simulink model "CommandLimits"  (R2017b)
settings: configuration reference "Autosar_CodeGeneration" (kept outside this file)
settings Model: RequirementInfo={'linktype_rmi_url' 'http://md1hxhhc.ww004.siemens.net/polarion/' '@/project/ATRover/workitem?id=ATR-529' 'true' 'Polarion: ATR-529' '' ; 'linktype_rmi_url' 'http://md1hxhhc.ww004.siemens.net/polarion/' '@/project/ATRover/workitem?id=ATR-594' 'true' 'Polarion: ATR-594' '' } %GIDa_e2c0a0a6_deb1_4459_85d0_b00cc8d3b9da  DataDictionary=RoverDataDict.sldd  Creator=zwqe6u  LastModifiedBy=eh6qym
settings ConfigSetRef: DDName=RoverDataDict.sldd

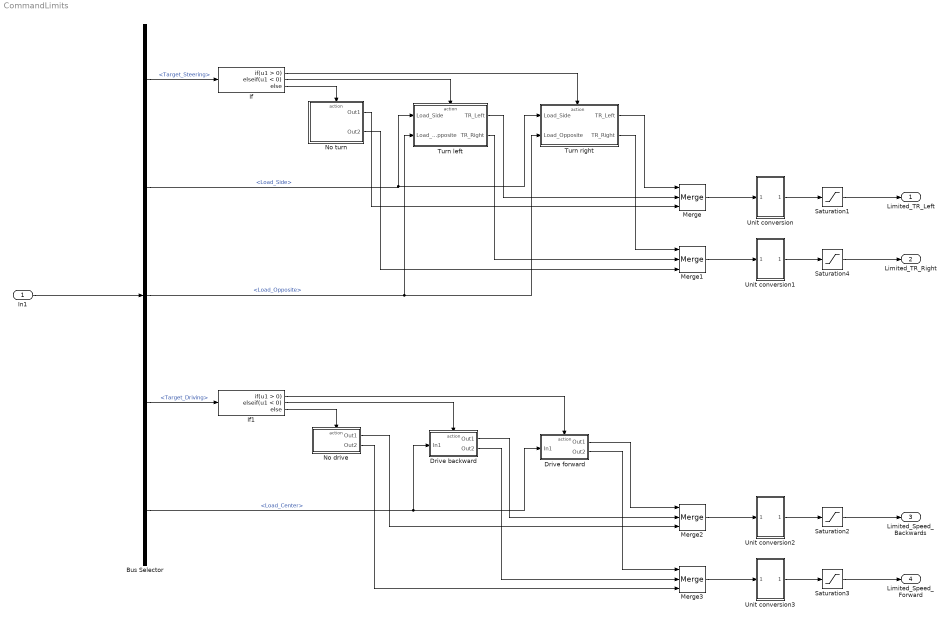
== system CommandLimits ==
  In1 : Inport  OutDataTypeStr=Bus: Obstacle_Detection_Out
  Bus Selector : BusSelector  OutputSignals=Target_Steering,Load_Side,Load_Opposite,Target_Driving,Load_Center
  Drive backward : Subsystem  TreatAsAtomicUnit=on
  Drive forward : Subsystem  TreatAsAtomicUnit=on
  If : If  ElseIfExpressions=u1 < 0
  If1 : If  ElseIfExpressions=u1 < 0
  Merge : Merge  Inputs=3  InitialOutput=[-1]
  Merge1 : Merge  Inputs=3  InitialOutput=[1]
  Merge2 : Merge  Inputs=3  InitialOutput=[-1]
  Merge3 : Merge  Inputs=3  InitialOutput=[1]
  No drive : Subsystem  TreatAsAtomicUnit=on
  No turn : Subsystem  TreatAsAtomicUnit=on
  Saturation1 : Saturate  UpperLimit=5  LowerLimit=0
  Saturation2 : Saturate  UpperLimit=2.5  LowerLimit=0
  Saturation3 : Saturate  UpperLimit=5  LowerLimit=2.5
  Saturation4 : Saturate  UpperLimit=5  LowerLimit=0
  Turn left : Subsystem  TreatAsAtomicUnit=on
  Turn right : Subsystem  TreatAsAtomicUnit=on
  Unit conversion : Subsystem
  Unit conversion1 : Subsystem
  Unit conversion2 : Subsystem
  Unit conversion3 : Subsystem
  Limited_TR_Left : Outport  OutDataTypeStr=double
  Limited_TR_Right : Outport  Port=2  OutDataTypeStr=double
  Limited_Speed_Backwards : Outport  Port=3  OutDataTypeStr=double
  Limited_Speed_Forward : Outport  Port=4  OutDataTypeStr=double
  wires:
  In1/1 -> Bus Selector/1
  Drive forward/1(Out1) -> Merge2/1
  Drive backward/1(Out1) -> Merge2/2
  Drive forward/2(Out2) -> Merge3/1
  Drive backward/2(Out2) -> Merge3/2
  Unit conversion2/1(Out1) -> Saturation2/1
  Unit conversion3/1(Out1) -> Saturation3/1
  Bus Selector/4 -> If1/1  "<Target_Driving>"
  If1/1 -> Drive forward/Action
  If1/2 -> Drive backward/Action
  Merge1/1 -> Unit conversion1/1(In1)
  Merge/1 -> Unit conversion/1(In1)
  Merge2/1 -> Unit conversion2/1(In1)
  Merge3/1 -> Unit conversion3/1(In1)
  Unit conversion/1(Out1) -> Saturation1/1
  Unit conversion1/1(Out1) -> Saturation4/1
  Saturation2/1 -> Limited_Speed_Backwards/1
  Saturation3/1 -> Limited_Speed_Forward/1
  Saturation1/1 -> Limited_TR_Left/1
  Saturation4/1 -> Limited_TR_Right/1
  If1/3 -> No drive/Action
  No drive/1(Out1) -> Merge2/3
  No drive/2(Out2) -> Merge3/3
  Bus Selector/5 -> Drive forward/1(In1), Drive backward/1(In1)  "<Load_Center>"
  Bus Selector/3 -> Turn right/2(Load_Opposite), Turn left/2(Load_Opposite)  "<Load_Opposite>"
  Bus Selector/2 -> Turn right/1(Load_Side), Turn left/1(Load_Side)  "<Load_Side>"
  Turn right/1(TR_Left) -> Merge/1
  Turn right/2(TR_Right) -> Merge1/1
  If/1 -> Turn right/Action
  If/2 -> Turn left/Action
  Turn left/1(TR_Left) -> Merge/2
  Turn left/2(TR_Right) -> Merge1/2
  If/3 -> No turn/Action
  No turn/1(Out1) -> Merge/3
  No turn/2(Out2) -> Merge1/3
  Bus Selector/1 -> If/1  "<Target_Steering>"

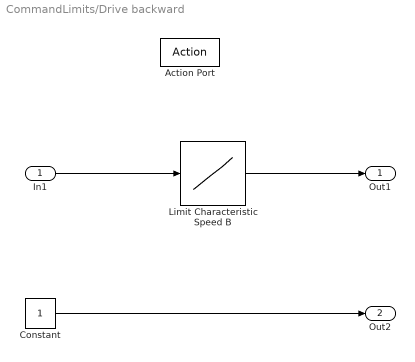
== system CommandLimits/Drive backward ==
  In1 : Inport
  Action Port : ActionPort  ActionType=elseif
  Constant : Constant
  Limit Characteristic Speed B : Lookup_n-D  NumberOfTableDimensions=1  BreakpointsForDimension1=[0.06 0.10 0.30 0.80]  Table=[0 0 -0.1 -1]  RemoveProtectionInput=on  InternalRulePriority=Speed  RndMeth=Simplest  InputSameDT=on
  Out1 : Outport  InitialOutput=[-1]
  Out2 : Outport  Port=2  InitialOutput=[1]
  wires:
  Limit Characteristic Speed B/1 -> Out1/1
  In1/1 -> Limit Characteristic Speed B/1
  Constant/1 -> Out2/1

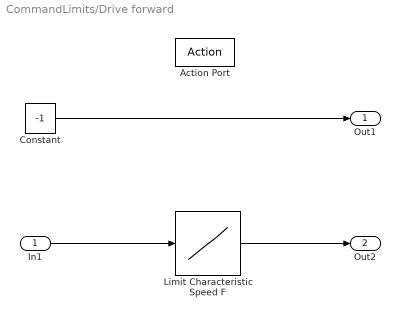
== system CommandLimits/Drive forward ==
  In1 : Inport
  Action Port : ActionPort  ActionType=then
  Constant : Constant  Value=-1
  Limit Characteristic Speed F : Lookup_n-D  NumberOfTableDimensions=1  BreakpointsForDimension1=[0.06 0.10 0.30 0.80]  Table=[0 0 0.1 1]  RemoveProtectionInput=on  InternalRulePriority=Speed  RndMeth=Simplest  InputSameDT=on
  Out1 : Outport  InitialOutput=[-1]
  Out2 : Outport  Port=2  InitialOutput=[1]
  wires:
  Limit Characteristic Speed F/1 -> Out2/1
  In1/1 -> Limit Characteristic Speed F/1
  Constant/1 -> Out1/1

== system CommandLimits/No drive ==
  Action Port : ActionPort  ActionType=else
  Constant : Constant  Value=-1
  Constant1 : Constant
  Out1 : Outport  InitialOutput=[0.8]
  Out2 : Outport  Port=2  InitialOutput=[0.8]
  wires:
  Constant/1 -> Out1/1
  Constant1/1 -> Out2/1

== system CommandLimits/No turn ==
  Action Port : ActionPort  ActionType=else
  Constant : Constant  Value=-1
  Constant1 : Constant
  Out1 : Outport  InitialOutput=[-1]
  Out2 : Outport  Port=2  InitialOutput=[1]
  wires:
  Constant/1 -> Out1/1
  Constant1/1 -> Out2/1

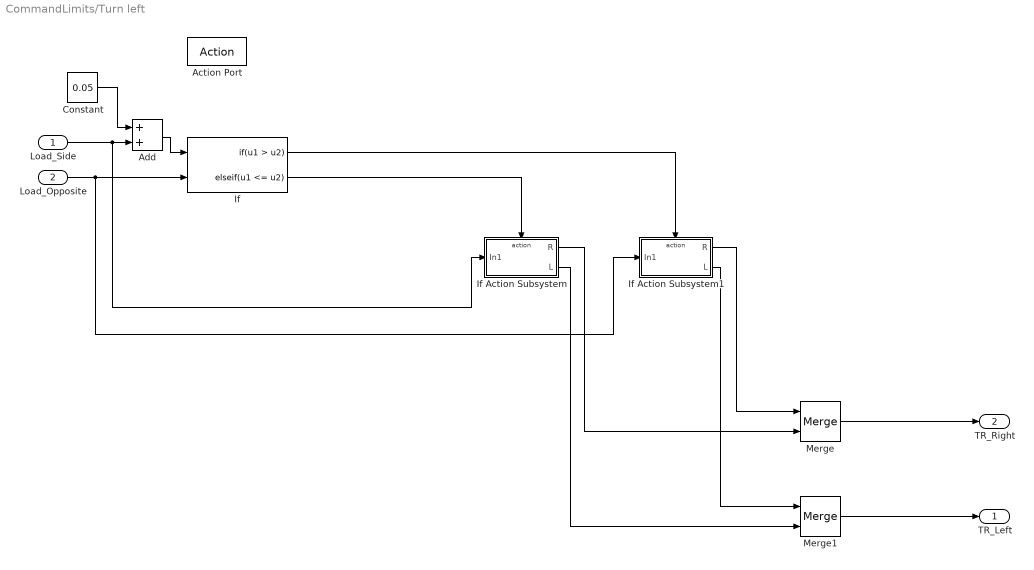
== system CommandLimits/Turn left ==
  Load_Side : Inport
  Load_Opposite : Inport  Port=2
  Action Port : ActionPort  ActionType=elseif
  Add : Sum
  Constant : Constant  Value=0.05
  If : If  NumInputs=2  IfExpression=u1 > u2  ElseIfExpressions=u1 <= u2  ShowElse=off
  If Action Subsystem : Subsystem  TreatAsAtomicUnit=on
  If Action Subsystem1 : Subsystem  TreatAsAtomicUnit=on
  Merge : Merge  InitialOutput=[1]
  Merge1 : Merge  InitialOutput=[-1]
  TR_Left : Outport  InitialOutput=[-1]
  TR_Right : Outport  Port=2  InitialOutput=[1]
  wires:
  Load_Opposite/1 -> If/2, If Action Subsystem1/1(In1)
  If Action Subsystem1/1(R) -> Merge/1
  If Action Subsystem/1(R) -> Merge/2
  If/1 -> If Action Subsystem1/Action
  If Action Subsystem/2(L) -> Merge1/2
  If Action Subsystem1/2(L) -> Merge1/1
  Load_Side/1 -> If Action Subsystem/1(In1), Add/2
  Merge1/1 -> TR_Left/1
  Merge/1 -> TR_Right/1
  If/2 -> If Action Subsystem/Action
  Constant/1 -> Add/1
  Add/1 -> If/1

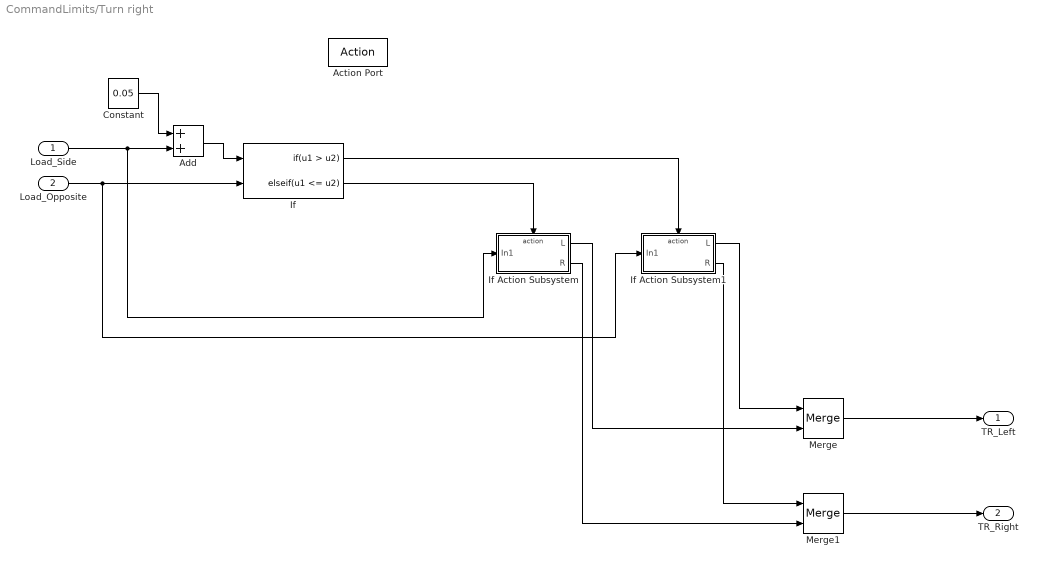
== system CommandLimits/Turn right ==
  Load_Side : Inport
  Load_Opposite : Inport  Port=2
  Action Port : ActionPort  ActionType=then
  Add : Sum
  Constant : Constant  Value=0.05
  If : If  NumInputs=2  IfExpression=u1 > u2  ElseIfExpressions=u1 <= u2  ShowElse=off
  If Action Subsystem : Subsystem  TreatAsAtomicUnit=on
  If Action Subsystem1 : Subsystem  TreatAsAtomicUnit=on
  Merge : Merge  InitialOutput=[-1]
  Merge1 : Merge  InitialOutput=[1]
  TR_Left : Outport  InitialOutput=[-1]
  TR_Right : Outport  Port=2  InitialOutput=[1]
  wires:
  Load_Opposite/1 -> If Action Subsystem1/1(In1), If/2
  If Action Subsystem1/1(L) -> Merge/1
  If Action Subsystem/1(L) -> Merge/2
  If/1 -> If Action Subsystem1/Action
  If Action Subsystem/2(R) -> Merge1/2
  Load_Side/1 -> Add/2, If Action Subsystem/1(In1)
  If Action Subsystem1/2(R) -> Merge1/1
  Merge/1 -> TR_Left/1
  Merge1/1 -> TR_Right/1
  If/2 -> If Action Subsystem/Action
  Add/1 -> If/1
  Constant/1 -> Add/1

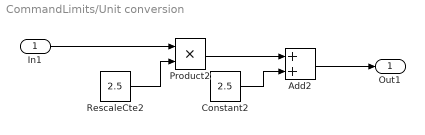
== system CommandLimits/Unit conversion ==
  In1 : Inport
  Add2 : Sum
  Constant2 : Constant  Value=2.5
  Product2 : Product
  RescaleCte2 : Constant  Value=2.5
  Out1 : Outport
  wires:
  RescaleCte2/1 -> Product2/2
  Constant2/1 -> Add2/2
  Add2/1 -> Out1/1
  Product2/1 -> Add2/1
  In1/1 -> Product2/1

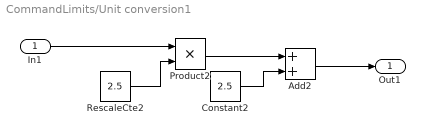
== system CommandLimits/Unit conversion1 ==
  In1 : Inport
  Add2 : Sum
  Constant2 : Constant  Value=2.5
  Product2 : Product
  RescaleCte2 : Constant  Value=2.5
  Out1 : Outport
  wires:
  RescaleCte2/1 -> Product2/2
  Constant2/1 -> Add2/2
  Add2/1 -> Out1/1
  Product2/1 -> Add2/1
  In1/1 -> Product2/1

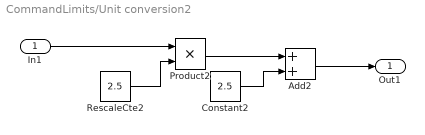
== system CommandLimits/Unit conversion2 ==
  In1 : Inport
  Add2 : Sum
  Constant2 : Constant  Value=2.5
  Product2 : Product
  RescaleCte2 : Constant  Value=2.5
  Out1 : Outport
  wires:
  RescaleCte2/1 -> Product2/2
  Constant2/1 -> Add2/2
  Add2/1 -> Out1/1
  Product2/1 -> Add2/1
  In1/1 -> Product2/1

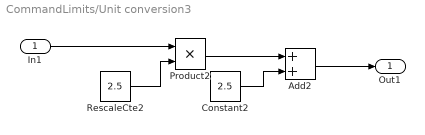
== system CommandLimits/Unit conversion3 ==
  In1 : Inport
  Add2 : Sum
  Constant2 : Constant  Value=2.5
  Product2 : Product
  RescaleCte2 : Constant  Value=2.5
  Out1 : Outport
  wires:
  RescaleCte2/1 -> Product2/2
  Constant2/1 -> Add2/2
  Add2/1 -> Out1/1
  Product2/1 -> Add2/1
  In1/1 -> Product2/1

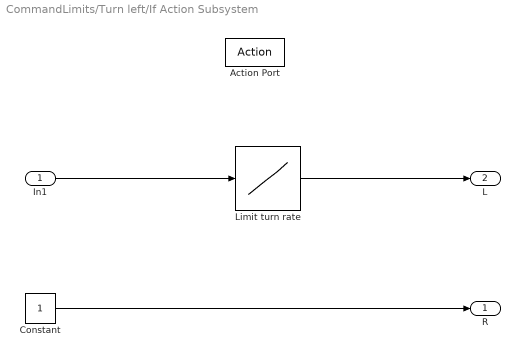
== system CommandLimits/Turn left/If Action Subsystem ==
  In1 : Inport
  Action Port : ActionPort  ActionType=elseif
  Constant : Constant
  Limit turn rate : Lookup_n-D  NumberOfTableDimensions=1  BreakpointsForDimension1=[0.06 0.5 0.8]  Table=[0.3 -0.8 -0.8]  RemoveProtectionInput=on  InternalRulePriority=Speed  RndMeth=Simplest  InputSameDT=on
  R : Outport  InitialOutput=[1]
  L : Outport  Port=2  InitialOutput=[-1]
  wires:
  Constant/1 -> R/1
  Limit turn rate/1 -> L/1
  In1/1 -> Limit turn rate/1

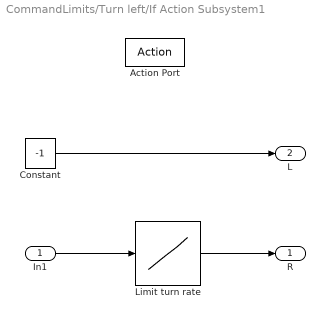
== system CommandLimits/Turn left/If Action Subsystem1 ==
  In1 : Inport
  Action Port : ActionPort  ActionType=then
  Constant : Constant  Value=-1
  Limit turn rate : Lookup_n-D  NumberOfTableDimensions=1  BreakpointsForDimension1=[0.06 0.8]  Table=[-0.3 0.8]  RemoveProtectionInput=on  InternalRulePriority=Speed  RndMeth=Simplest  InputSameDT=on
  R : Outport  InitialOutput=[-0.5]
  L : Outport  Port=2  InitialOutput=[-1]
  wires:
  In1/1 -> Limit turn rate/1
  Constant/1 -> L/1
  Limit turn rate/1 -> R/1

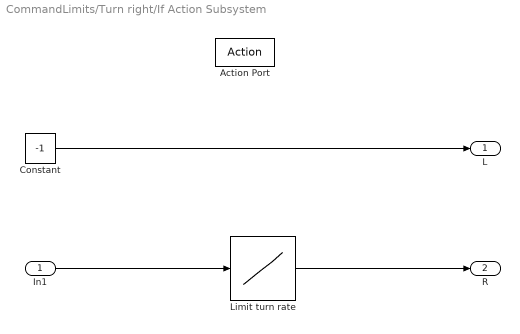
== system CommandLimits/Turn right/If Action Subsystem ==
  In1 : Inport
  Action Port : ActionPort  ActionType=elseif
  Constant : Constant  Value=-1
  Limit turn rate : Lookup_n-D  NumberOfTableDimensions=1  BreakpointsForDimension1=[0.06 0.5 0.8]  Table=[-0.3 0.8 0.8]  RemoveProtectionInput=on  InternalRulePriority=Speed  RndMeth=Simplest  InputSameDT=on
  L : Outport  InitialOutput=[-1]
  R : Outport  Port=2  InitialOutput=[1]
  wires:
  Constant/1 -> L/1
  Limit turn rate/1 -> R/1
  In1/1 -> Limit turn rate/1

== system CommandLimits/Turn right/If Action Subsystem1 ==
  In1 : Inport
  Action Port : ActionPort  ActionType=then
  Constant : Constant
  Limit turn rate : Lookup_n-D  NumberOfTableDimensions=1  BreakpointsForDimension1=[0.06 0.8]  Table=[0.3 -0.8]  RemoveProtectionInput=on  InternalRulePriority=Speed  RndMeth=Simplest  InputSameDT=on
  L : Outport  InitialOutput=[0.01]
  R : Outport  Port=2  InitialOutput=[1]
  wires:
  Constant/1 -> R/1
  Limit turn rate/1 -> L/1
  In1/1 -> Limit turn rate/1
